simulink model "model"  (R2024b)
settings: Solver=VariableStepAuto  StartTime=0.0  StopTime=20  RelTol=1e-3
values from neighbouring files (symbols this model uses):
  a = 0.01    [zad2_params.m]
  alpha = 0.5    [zad3_params.m]
  beta = 1    [zad3_params.m]
  K = 0.5    [zad3_params.m]
  k = 0.5    [zad2_params.m]
  m = 1    [zad2_params.m]
settings Model: Creator=student  LastModifiedBy=SzymonWysoglad
settings RTWCC: GPUComputeCapability=3.5

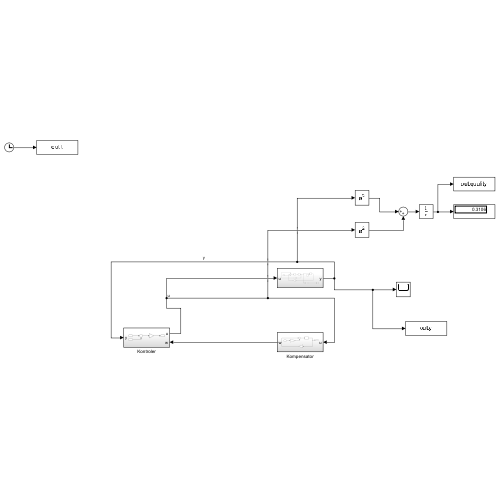
[thumbnail: Simulink's stored preview of the top-level diagram]
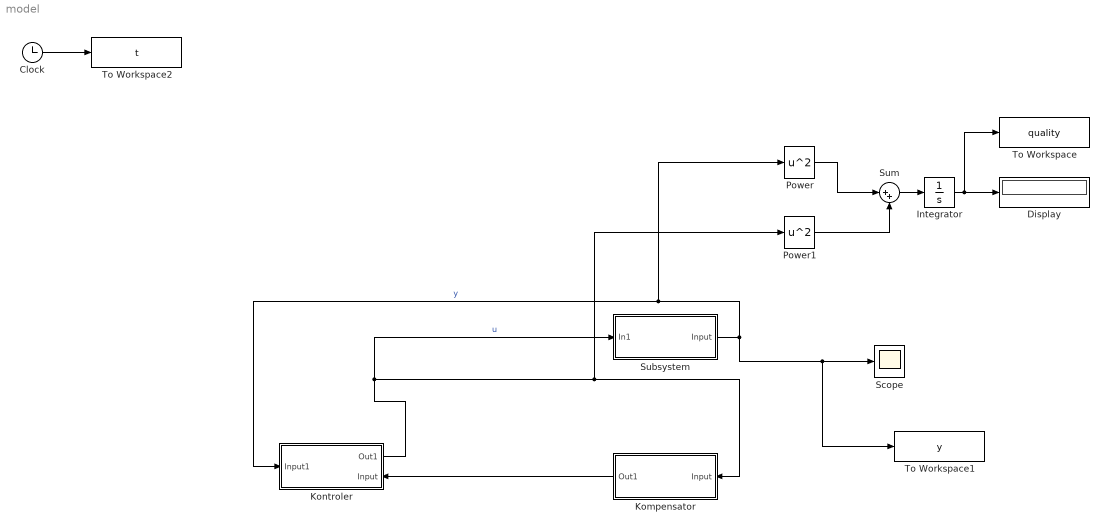
== system model ==
  Clock : Clock
  Display : Display
  Integrator : Integrator
  Kompensator : Subsystem
      settings: PortSchema="{\"entries\":[{\"content\":{\"sides\":[{\"content\":{\"connectorIds\":[\"Out1\"]},\"type\":\"ConnectorPlacement.EquallySpacedRectSide\",\"uuid\":\"271025cb-5b0e-4eb0-b2bb-185f6bd932cc\"},{\"content\":{\"connectorIds\":[\"In1\"],\"side\":\"RIGHT\"},\"type\":\"ConnectorPlacement.EquallySpacedRectSide\",\"uuid\":\"bf34e8a7-b6c3-40dc-9974-43b0fd2d3e9b\"},{\"content\":{\"side\":\"TOP\"},\"type\":\"ConnectorPlacement.EquallySpacedRectSide\",\"uuid\":\"8ac63cdf-fd16-4648-a61e-dba41989f7d6\"}]},\"type\":\"ConnectorPlacement.EquallySpacedConnector\",\"uuid\":\"20f92b2e-def0-4c6b-b1a1-a655338ea2f6\"}],\"packageUris\":[\"http://schema.mathworks.com/mf0/Connector/R2020b\"],\"version\":\"1.0\"}"
  Kontroler : Subsystem
      settings: PortSchema="{\"entries\":[{\"content\":{\"sides\":[{\"content\":{\"connectorIds\":[\"In1\"]},\"type\":\"ConnectorPlacement.EquallySpacedRectSide\",\"uuid\":\"1ab95de1-d027-4ffa-837b-20cb4805244c\"},{\"content\":{\"connectorIds\":[\"Out1\",\"In2\"],\"side\":\"RIGHT\"},\"type\":\"ConnectorPlacement.EquallySpacedRectSide\",\"uuid\":\"ae6915cd-01ca-4123-b107-ec52aab3fbe3\"},{\"content\":{\"side\":\"TOP\"},\"type\":\"ConnectorPlacement.EquallySpacedRectSide\",\"uuid\":\"9f47001c-baf8-42b9-ba39-d9622ca83bc8\"}]},\"type\":\"ConnectorPlacement.EquallySpacedConnector\",\"uuid\":\"f0a290e3-0f19-4760-b900-1ff6d9b147f3\"}],\"packageUris\":[\"http://schema.mathworks.com/mf0/Connector/R2020b\"],\"version\":\"1.0\"}"
  Power : Math  Operator=square
  Power1 : Math  Operator=square
  Scope : Scope
  Subsystem : Subsystem
  Sum : Sum  Inputs=|++
  To Workspace : ToWorkspace  VariableName=quality  SampleTime=-1
  To Workspace1 : ToWorkspace  VariableName=y  SampleTime=-1
  To Workspace2 : ToWorkspace  VariableName=t  SampleTime=-1
  wires:
  Subsystem/1(Input) -> Power/1, Kontroler/1(Input1), To Workspace1/1, Scope/1  "y"
  Kontroler/1(Out1) -> Subsystem/1(In1), Power1/1, Kompensator/1(Input)  "u"
  Kompensator/1(Out1) -> Kontroler/2(Input)
  Power/1 -> Sum/1
  Power1/1 -> Sum/2
  Sum/1 -> Integrator/1
  Integrator/1 -> Display/1, To Workspace/1
  Clock/1 -> To Workspace2/1

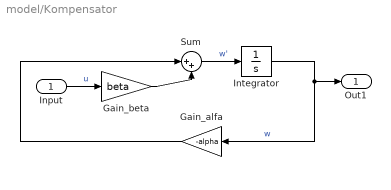
== system model/Kompensator ==
  Input : Inport
  Gain_alfa : Gain  Gain=-alpha
  Gain_beta : Gain  Gain=beta
  Integrator : Integrator
  Sum : Sum  Inputs=|++
  Out1 : Outport
  wires:
  Sum/1 -> Integrator/1  "w'"
  Gain_alfa/1 -> Sum/1
  Integrator/1 -> Gain_alfa/1, Out1/1  "w"
  Gain_beta/1 -> Sum/2
  Input/1 -> Gain_beta/1  "u"

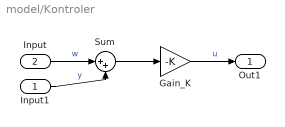
== system model/Kontroler ==
  Input1 : Inport
  Input : Inport  Port=2
  Gain_K : Gain  Gain=-K
  Sum : Sum  Inputs=|++
  Out1 : Outport
  wires:
  Gain_K/1 -> Out1/1  "u"
  Input/1 -> Sum/1  "w"
  Input1/1 -> Sum/2  "y"
  Sum/1 -> Gain_K/1

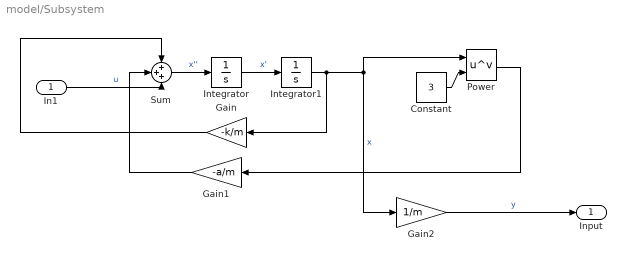
== system model/Subsystem ==
  In1 : Inport
  Constant : Constant  Value=3
  Gain : Gain  Gain=-k/m
  Gain1 : Gain  Gain=-a/m
  Gain2 : Gain  Gain=1/m
  Integrator : Integrator
  Integrator1 : Integrator  InitialCondition=0.5
  Power : Math  Operator=pow
  Sum : Sum  Inputs=+++
  Input : Outport
  wires:
  Gain2/1 -> Input/1  "y"
  Power/1 -> Gain1/1
  Gain1/1 -> Sum/2
  Integrator1/1 -> Gain/1, Power/1, Gain2/1  "x"
  Sum/1 -> Integrator/1  "x''"
  Gain/1 -> Sum/1
  Integrator/1 -> Integrator1/1  "x'"
  In1/1 -> Sum/3  "u"
  Constant/1 -> Power/2
